simulink model "flocking_algorithm"  (R2025b)
settings: Solver=ode4  StartTime=0.0  StopTime=500  FixedStep=0.01  RelTol=1e-3
libraries: simulink_extras x9
(part 1 of 2)
settings Model: Creator=chang  LastModifiedBy=Administrator

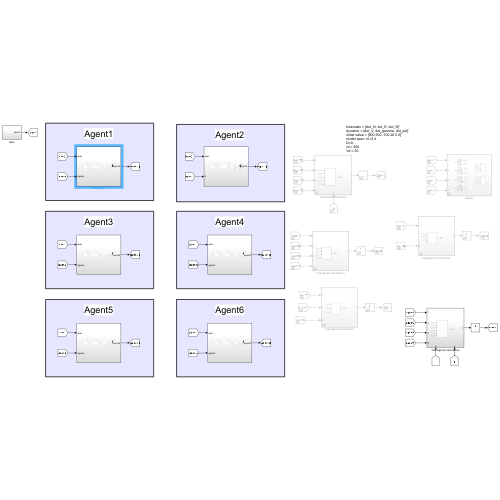
[thumbnail: Simulink's stored preview of the top-level diagram]
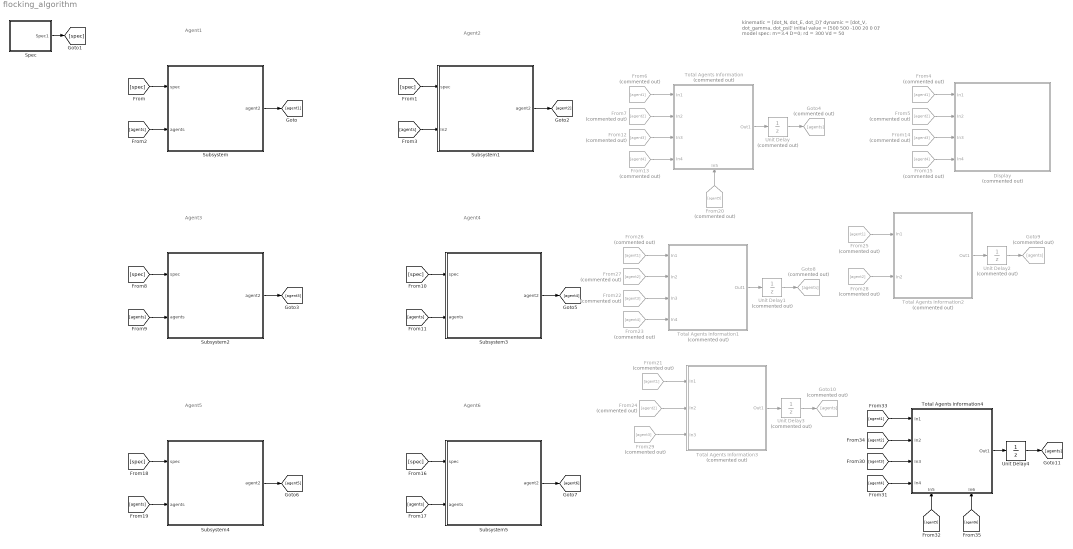
== system flocking_algorithm ==
  note: Agent1
  note: kinematic = [dot_N, dot_E, dot_D]'
      | dynamic = [dot_V, dot_gamma, dot_psi]'
      | initial value = [500 500 -100 20 0 0]'
      | model spec: m=3.4
      | D=0;
      | rd = 300
      | Vd = 50
  note: Agent2
  note: Agent3
  note: Agent4
  note: Agent5
  note: Agent6
  Display : Subsystem  Commented=on
  From{12,14,22,29} (4 alike) : From  Commented=on  GotoTag=agent3
  From13 : From  Commented=on  GotoTag=agent4
  From15 : From  Commented=on  GotoTag=agent4
  From20 : From  Commented=on  GotoTag=agent5
  From{4,6,21,25..26} (5 alike) : From  Commented=on  GotoTag=agent1
  From23 : From  Commented=on  GotoTag=agent4
  From{5,7,24,27..28} (5 alike) : From  Commented=on  GotoTag=agent2
  Goto{4,8..10} (4 alike) : Goto  Commented=on  GotoTag=agents
  Spec : Subsystem
  Subsystem : Subsystem
  Subsystem1 : Subsystem
  Subsystem2 : Subsystem
  Subsystem3 : Subsystem
  Subsystem4 : Subsystem
  Subsystem5 : Subsystem
  Total Agents Information : Subsystem  Commented=on
      settings: PortSchema="{\"entries\":[{\"content\":{\"sides\":[{\"content\":{\"connectorIds\":[\"In1\",\"In2\",\"In3\",\"In4\"]},\"type\":\"ConnectorPlacement.EquallySpacedRectSide\",\"uuid\":\"e43ed8c9-8aa1-4204-b6a6-30ae9222babf\"},{\"content\":{\"connectorIds\":[\"Out1\"],\"side\":\"RIGHT\"},\"type\":\"ConnectorPlacement.EquallySpacedRectSide\",\"uuid\":\"08aef384-d870-4c51-a80b-184b5836c24d\"},{\"content\":{\"side\":\"TOP\"},\"type\":\"ConnectorPlacement.EquallySpacedRectSide\",\"uuid\":\"5ba70bed-f88c-44da-8fba-8008d18066d7\"},{\"content\":{\"connectorIds\":[\"In5\"],\"side\":\"BOTTOM\"},\"type\":\"ConnectorPlacement.EquallySpacedRectSide\",\"uuid\":\"c2369018-f13e-4eb4-997b-0da9921f82e2\"}]},\"type\":\"ConnectorPlacement.EquallySpacedConnector\",\"uuid\":\"929a7d50-5615-46ab-b178-754a3aebd756\"}],\"packageUris\":[\"http://schema.mathworks.com/mf0/Connector/R2020b\"],\"version\":\"1.0\"}"
  Total Agents Information1 : Subsystem  Commented=on
  Total Agents Information2 : Subsystem  Commented=on
  Total Agents Information3 : Subsystem  Commented=on
  Total Agents Information4 : Subsystem
      settings: PortSchema="{\"entries\":[{\"content\":{\"sides\":[{\"content\":{\"connectorIds\":[\"In1\",\"In2\",\"In3\",\"In4\"]},\"type\":\"ConnectorPlacement.EquallySpacedRectSide\",\"uuid\":\"e43ed8c9-8aa1-4204-b6a6-30ae9222babf\"},{\"content\":{\"connectorIds\":[\"Out1\"],\"side\":\"RIGHT\"},\"type\":\"ConnectorPlacement.EquallySpacedRectSide\",\"uuid\":\"08aef384-d870-4c51-a80b-184b5836c24d\"},{\"content\":{\"side\":\"TOP\"},\"type\":\"ConnectorPlacement.EquallySpacedRectSide\",\"uuid\":\"5ba70bed-f88c-44da-8fba-8008d18066d7\"},{\"content\":{\"connectorIds\":[\"In5\",\"In6\"],\"side\":\"BOTTOM\"},\"type\":\"ConnectorPlacement.EquallySpacedRectSide\",\"uuid\":\"c2369018-f13e-4eb4-997b-0da9921f82e2\"}]},\"type\":\"ConnectorPlacement.EquallySpacedConnector\",\"uuid\":\"929a7d50-5615-46ab-b178-754a3aebd756\"}],\"packageUris\":[\"http://schema.mathworks.com/mf0/Connector/R2020b\"],\"version\":\"1.0\"}"
  Unit Delay{,1..3} (4 alike) : UnitDelay  Commented=on  SampleTime=-1  HasFrameUpgradeWarning=on
  Unit Delay4 : UnitDelay  SampleTime=-1  HasFrameUpgradeWarning=on
  wires:
  [spec] -> Subsystem/1(spec)
  [agents] -> Subsystem/2(agents)
  Subsystem1/1(agent2) -> [agent2]
  [agents] -> Subsystem1/2(In2)
  [spec] -> Subsystem1/1(spec)
  Subsystem/1(agent2) -> [agent1]
  Spec/1(Spec1) -> [spec]
  Unit Delay/1 -> Goto4/1
  From4/1 -> Display/1(In1)
  From5/1 -> Display/2(In2)
  From6/1 -> Total Agents Information/1(In1)
  From7/1 -> Total Agents Information/2(In2)
  Total Agents Information/1(Out1) -> Unit Delay/1
  [spec] -> Subsystem2/1(spec)
  [agents] -> Subsystem2/2(agents)
  Subsystem2/1(agent2) -> [agent3]
  [spec] -> Subsystem3/1(spec)
  [agents] -> Subsystem3/2(agents)
  Subsystem3/1(agent2) -> [agent4]
  From12/1 -> Total Agents Information/3(In3)
  From13/1 -> Total Agents Information/4(In4)
  From15/1 -> Display/4(In4)
  From14/1 -> Display/3(In3)
  [spec] -> Subsystem4/1(spec)
  [agents] -> Subsystem4/2(agents)
  [spec] -> Subsystem5/1(spec)
  Subsystem5/1(agent2) -> [agent6]
  [agents] -> Subsystem5/2(agents)
  Subsystem4/1(agent2) -> [agent5]
  From20/1 -> Total Agents Information/5(In5)
  Unit Delay1/1 -> Goto8/1
  From27/1 -> Total Agents Information1/2(In2)
  Total Agents Information1/1(Out1) -> Unit Delay1/1
  From26/1 -> Total Agents Information1/1(In1)
  From22/1 -> Total Agents Information1/3(In3)
  From23/1 -> Total Agents Information1/4(In4)
  From25/1 -> Total Agents Information2/1(In1)
  Unit Delay2/1 -> Goto9/1
  From28/1 -> Total Agents Information2/2(In2)
  Total Agents Information2/1(Out1) -> Unit Delay2/1
  From24/1 -> Total Agents Information3/2(In2)
  Unit Delay3/1 -> Goto10/1
  From21/1 -> Total Agents Information3/1(In1)
  Total Agents Information3/1(Out1) -> Unit Delay3/1
  From29/1 -> Total Agents Information3/3(In3)
  [agent5] -> Total Agents Information4/5(In5)
  Total Agents Information4/1(Out1) -> Unit Delay4/1
  Unit Delay4/1 -> [agents]
  [agent2] -> Total Agents Information4/2(In2)
  [agent1] -> Total Agents Information4/1(In1)
  [agent3] -> Total Agents Information4/3(In3)
  [agent4] -> Total Agents Information4/4(In4)
  [agent6] -> Total Agents Information4/6(In6)

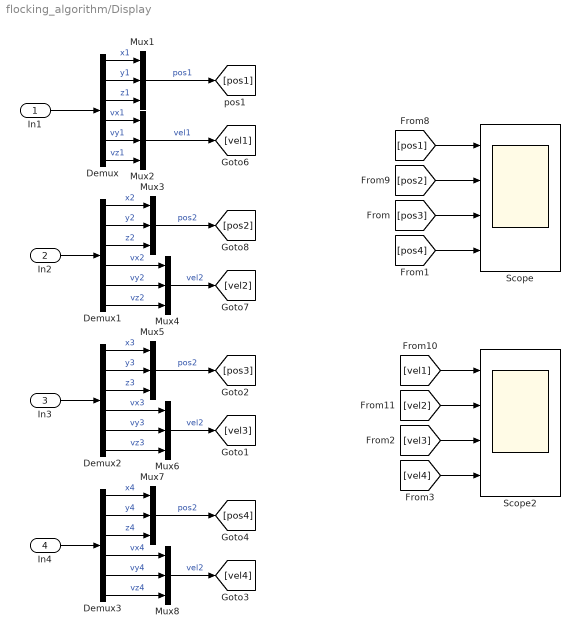
== system flocking_algorithm/Display ==
  In1 : Inport
  In2 : Inport  Port=2
  In3 : Inport  Port=3
  In4 : Inport  Port=4
  Demux{,1..3} (4 alike) : Demux  Outputs=6
  Mux{1..8} (8 alike) : Mux  Inputs=3
  Scope : Scope  NumInputPorts=4
      settings: ActiveDisplayYMinimum=-791.01816561476244  ActiveDisplayYMaximum=1093.5677488237882
  Scope2 : Scope  NumInputPorts=4
      settings: ActiveDisplayYMinimum=-365.07848233983896  ActiveDisplayYMaximum=72.840870211825987  DataLoggingVariableName=ScopeData7
  wires:
  Mux3/1 -> [pos2]  "pos2"
  Demux1/4 -> Mux4/1  "vx2"
  [pos2] -> Scope/2
  Demux/6 -> Mux2/3  "vz1"
  Demux/1 -> Mux1/1  "x1"
  Demux/4 -> Mux2/1  "vx1"
  Demux1/5 -> Mux4/2  "vy2"
  Mux2/1 -> [vel1]  "vel1"
  [vel1] -> Scope2/1
  Demux1/2 -> Mux3/2  "y2"
  Demux/3 -> Mux1/3  "z1"
  Demux/2 -> Mux1/2  "y1"
  Demux1/1 -> Mux3/1  "x2"
  Demux1/3 -> Mux3/3  "z2"
  [pos1] -> Scope/1
  Mux4/1 -> [vel2]  "vel2"
  Demux1/6 -> Mux4/3  "vz2"
  Mux1/1 -> [pos1]  "pos1"
  Demux/5 -> Mux2/2  "vy1"
  [vel2] -> Scope2/2
  In2/1 -> Demux1/1
  In1/1 -> Demux/1
  Demux2/5 -> Mux6/2  "vy3"
  Demux2/6 -> Mux6/3  "vz3"
  Demux2/4 -> Mux6/1  "vx3"
  Mux5/1 -> [pos3]  "pos2"
  In3/1 -> Demux2/1
  Demux2/3 -> Mux5/3  "z3"
  Mux6/1 -> [vel3]  "vel2"
  Demux2/1 -> Mux5/1  "x3"
  Demux2/2 -> Mux5/2  "y3"
  Demux3/5 -> Mux8/2  "vy4"
  Demux3/6 -> Mux8/3  "vz4"
  Demux3/4 -> Mux8/1  "vx4"
  Mux7/1 -> [pos4]  "pos2"
  In4/1 -> Demux3/1
  Demux3/3 -> Mux7/3  "z4"
  Mux8/1 -> [vel4]  "vel2"
  Demux3/1 -> Mux7/1  "x4"
  Demux3/2 -> Mux7/2  "y4"
  [pos3] -> Scope/3
  [pos4] -> Scope/4
  [vel3] -> Scope2/3
  [vel4] -> Scope2/4

== system flocking_algorithm/Spec ==
  Spec : Subsystem
  Spec1 : Outport
  wires:
  Spec/1(Spec) -> Spec1/1

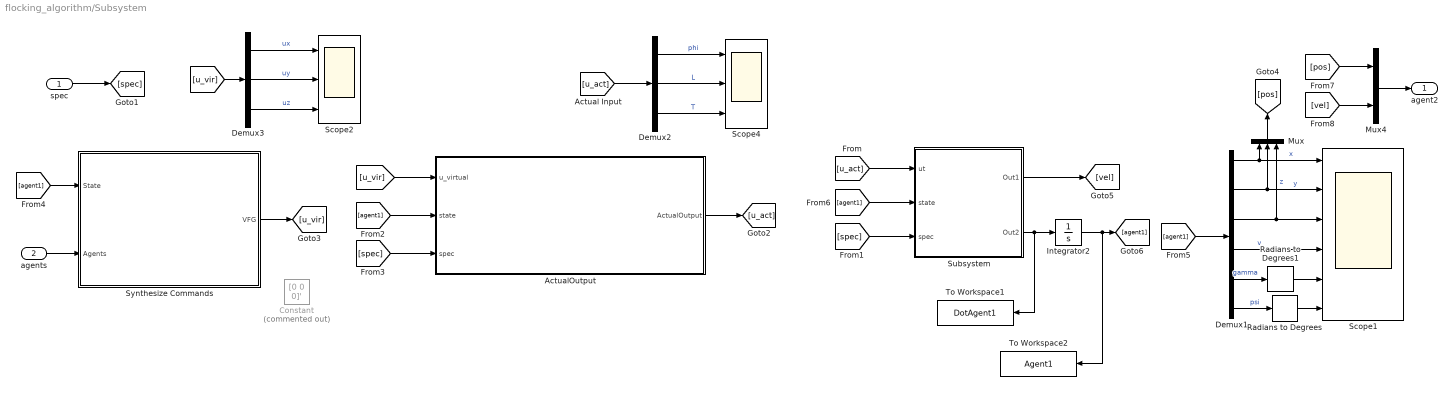
== system flocking_algorithm/Subsystem ==
  spec : Inport
  agents : Inport  Port=2
  ActualOutput : Subsystem
  Constant : Constant  Commented=on  Value=[0 0 0]'
  Demux1 : Demux  Outputs=6
  Demux2 : Demux  Outputs=3
  Demux3 : Demux  Outputs=3
  Integrator2 : Integrator  InitialCondition=[-1800 2000 -100 20 0 0]'  UpperSaturationLimit=[10^6 ;10^6 ;10^6 ;30 ;15 ;10^6]  LowerSaturationLimit=[-10^6; -10^6 ;-10^6; 0; -15 ;-10^6]'
  Mux : Mux  Inputs=3
  Mux4 : Mux  Inputs=2
  Radians to Degrees : simulink_extras/Transformations/Radians to Degrees
  Radians to Degrees1 : simulink_extras/Transformations/Radians to Degrees
  Scope1 : Scope  NumInputPorts=6
      settings: ActiveDisplayYMinimum=-1.7966158577892821E+72  ActiveDisplayYMaximum=1.5570735154634757E+73  DataLoggingVariableName=ScopeData3
  Scope2 : Scope  NumInputPorts=3
      settings: ActiveDisplayYMinimum=-5.0247050713987121E+98  ActiveDisplayYMaximum=6.7419493762501636E+97
  Scope4 : Scope  NumInputPorts=3
      settings: ActiveDisplayYMinimum=-3.9266304802667316  ActiveDisplayYMaximum=3.9246740137432026  DataLoggingVariableName=ScopeData5
  Subsystem : Subsystem
  Synthesize Commands : Subsystem
  To Workspace1 : ToWorkspace  VariableName=DotAgent1  SaveFormat=Timeseries  SampleTime=-1
  To Workspace2 : ToWorkspace  VariableName=Agent1  SaveFormat=Timeseries  SampleTime=-1
  agent2 : Outport
  wires:
  [agent1] -> ActualOutput/2(state)
  Demux1/3 -> Mux/3, Scope1/3  "z"
  Demux1/4 -> Scope1/4  "v"
  Demux1/1 -> Mux/1, Scope1/1  "x"
  [spec] -> ActualOutput/3(spec)
  Demux2/1 -> Scope4/1  "phi"
  Demux2/3 -> Scope4/3  "T"
  Demux1/2 -> Mux/2, Scope1/2  "y"
  Demux2/2 -> Scope4/2  "L"
  [u_vir] -> Demux3/1
  [agent1] -> Demux1/1
  Demux1/5 -> Radians to Degrees1/1  "gamma"
  Demux1/6 -> Radians to Degrees/1  "psi"
  [u_act] -> Demux2/1
  Demux3/2 -> Scope2/2  "uy"
  Demux3/1 -> Scope2/1  "ux"
  Demux3/3 -> Scope2/3  "uz"
  [u_vir] -> ActualOutput/1(u_virtual)
  spec/1 -> [spec]
  Mux/1 -> [pos]
  Integrator2/1 -> [agent1], To Workspace2/1
  Mux4/1 -> agent2/1
  [vel] -> Mux4/2
  [pos] -> Mux4/1
  [agent1] -> Synthesize Commands/1(State)
  agents/1 -> Synthesize Commands/2(Agents)
  [u_act] -> Subsystem/1(ut)
  [agent1] -> Subsystem/2(state)
  [spec] -> Subsystem/3(spec)
  Subsystem/1(Out1) -> [vel]
  Subsystem/2(Out2) -> To Workspace1/1, Integrator2/1
  Synthesize Commands/1(VFG) -> [u_vir]
  ActualOutput/1(ActualOutput) -> [u_act]
  Radians to Degrees/1 -> Scope1/6
  Radians to Degrees1/1 -> Scope1/5

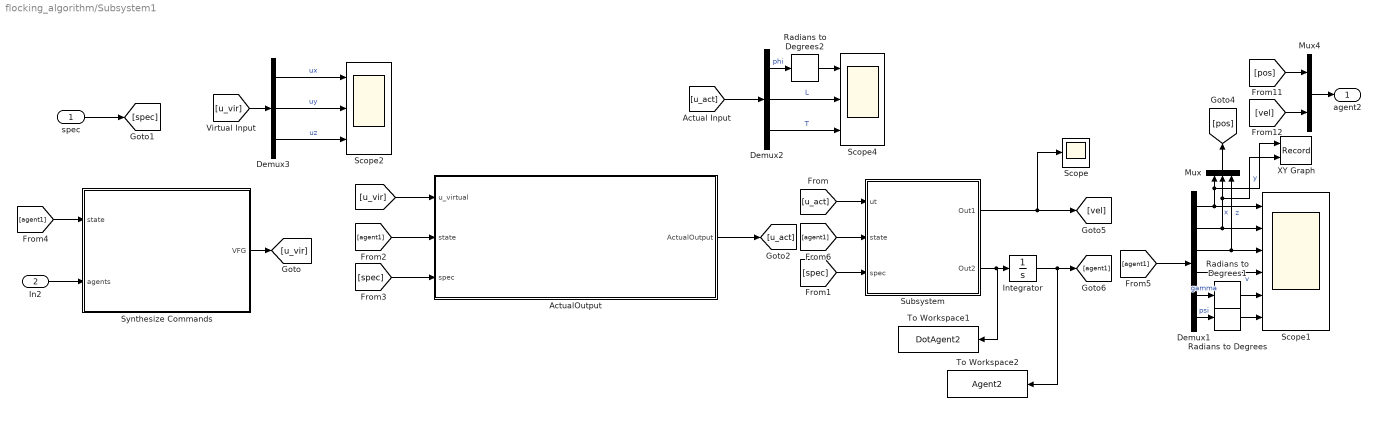
== system flocking_algorithm/Subsystem1 ==
  spec : Inport
  In2 : Inport  Port=2
  ActualOutput : Subsystem
  Demux1 : Demux  Outputs=6
  Demux2 : Demux  Outputs=3
  Demux3 : Demux  Outputs=3
  Integrator : Integrator  InitialCondition=[2000 1800 -100 20 0 0]'
  Mux : Mux  Inputs=3
  Mux4 : Mux  Inputs=2
  Radians to Degrees : simulink_extras/Transformations/Radians to Degrees
  Radians to Degrees1 : simulink_extras/Transformations/Radians to Degrees
  Radians to Degrees2 : simulink_extras/Transformations/Radians to Degrees
  Scope : Scope
      settings: ActiveDisplayYMinimum=-24.999999982546566  ActiveDisplayYMaximum=24.99999999806073  DataLoggingVariableName=ScopeData9
  Scope1 : Scope  NumInputPorts=6
      settings: ActiveDisplayYMinimum=-752.136140008936  ActiveDisplayYMaximum=1201.12192036178  DataLoggingVariableName=ScopeData3
  Scope2 : Scope  NumInputPorts=3
      settings: ActiveDisplayYMinimum=-50.131614103473233  ActiveDisplayYMaximum=7.8433072052775152
  Scope4 : Scope  NumInputPorts=3
      settings: ActiveDisplayYMinimum=-114.79277060053131  ActiveDisplayYMaximum=208.28266105424055  DataLoggingVariableName=ScopeData5
  Subsystem : Subsystem
  Synthesize Commands : Subsystem
  To Workspace1 : ToWorkspace  VariableName=DotAgent2  SaveFormat=Timeseries  SampleTime=-1
  To Workspace2 : ToWorkspace  VariableName=Agent2  SaveFormat=Timeseries  SampleTime=-1
  XY Graph : Record  NumPorts=2.0  FileSettingsInternal="{\"entries\":[{\"content\":{\"excelSettings\":{\"content\":{},\"type\":\"Streamout.ExcelSettings\"},\"parquetSettings\":{\"content\":{},\"type\":\"Streamout.ParquetSettings\"}},\"type\":\"Streamout.FileSettingStorage\",\"uuid\":\"\"}],\"packageUris\":[\"http:\\/\\/schema.mathworks.com\\/mf0\\/streamout_blocks\\/R2020a\"],\"version\":\"1.0\"}"  FrameSettings=[0, 0]  Layout=[1 1]  SignalsInternal="{\"entries\":[{\"content\":{\"signals\":[{\"content\":{\"blockPath\":[],\"dimensions\":[1],\"domain\":\"\",\"lineColor\":\"#a2142f\",\"plots\":[ 1 ],\"port\":1,\"signalID\":1,\"signalName\":\"x\"},\"type\":\"RecordBlkView.Signal\",\"uuid\":\"\"},{\"content\":{\"blockPath\":[],\"dimensions\":[1],\"domain\":\"\",\"lineColor\":\"#139fff\",\"plots\":[ 1 ],\"port\":2,\"signalID\":2,\"signalName\":\"y\"},\"type\":\"RecordBlkView.Signal\",\"uuid\":\"\"}]},\"type\":\"RecordBlkView.InputSignals\",\"uuid\":\"\"}],\"packageUris\":[\"http:\\/\\/schema.mathworks.com\\/mf0\\/streamout_blocks\\/R2020a\"],\"version\":\"1.0\"}"  VisualizationBindings="{\"xyplotplugin\":{\"info\":[{\"series\":[{\"bindingParametersList\":[{\"parameter\":\"X-Axis\",\"signalID\":1,\"signalName\":\"x\"},{\"parameter\":\"Y-Axis\",\"signalID\":2,\"signalName\":\"y\"}],\"seriesID\":0}],\"subplotID\":1}]}}"  CompatibilityTag=XY
  agent2 : Outport
  wires:
  [agent1] -> ActualOutput/2(state)
  Demux1/3 -> Scope1/3, Mux/3  "z"
  Demux1/4 -> Scope1/4  "v"
  Demux1/1 -> Scope1/1, XY Graph/1, Mux/1  "x"
  [spec] -> ActualOutput/3(spec)
  ActualOutput/1(ActualOutput) -> [u_act]
  Demux2/1 -> Radians to Degrees2/1  "phi"
  Demux2/3 -> Scope4/3  "T"
  Demux1/2 -> Scope1/2, XY Graph/2, Mux/2  "y"
  Demux2/2 -> Scope4/2  "L"
  [u_vir] -> Demux3/1
  [agent1] -> Demux1/1
  Demux1/5 -> Radians to Degrees1/1  "gamma"
  Demux1/6 -> Radians to Degrees/1  "psi"
  [u_act] -> Demux2/1
  Demux3/2 -> Scope2/2  "uy"
  Demux3/1 -> Scope2/1  "ux"
  Demux3/3 -> Scope2/3  "uz"
  [u_vir] -> ActualOutput/1(u_virtual)
  spec/1 -> [spec]
  Mux/1 -> [pos]
  [pos] -> Mux4/1
  [vel] -> Mux4/2
  Mux4/1 -> agent2/1
  Subsystem/2(Out2) -> To Workspace1/1, Integrator/1
  [agent1] -> Synthesize Commands/1(state)
  Synthesize Commands/1(VFG) -> [u_vir]
  [u_act] -> Subsystem/1(ut)
  [agent1] -> Subsystem/2(state)
  [spec] -> Subsystem/3(spec)
  Subsystem/1(Out1) -> Scope/1, [vel]
  Radians to Degrees/1 -> Scope1/6
  Radians to Degrees1/1 -> Scope1/5
  Radians to Degrees2/1 -> Scope4/1
  In2/1 -> Synthesize Commands/2(agents)
  Integrator/1 -> [agent1], To Workspace2/1

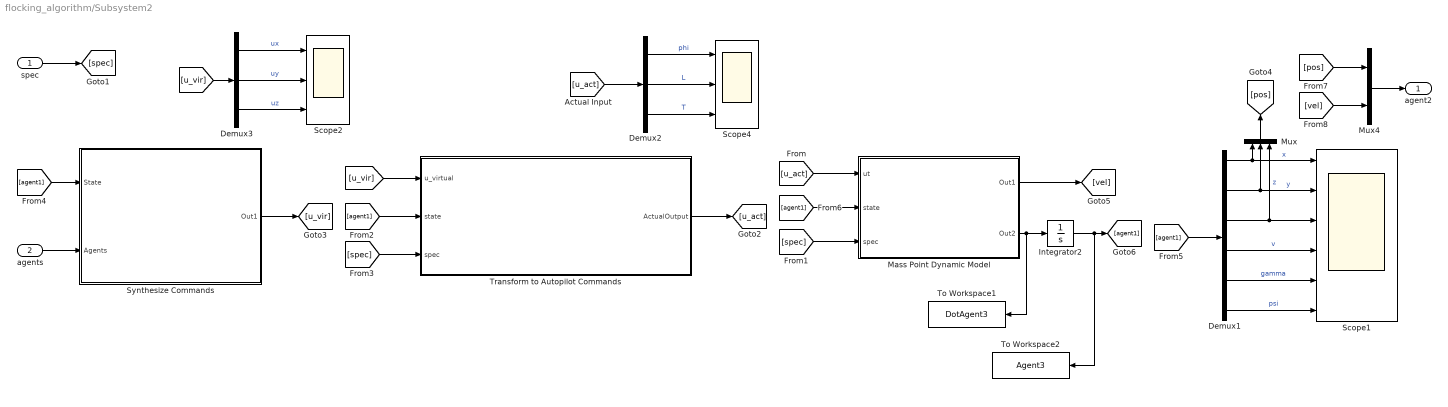
== system flocking_algorithm/Subsystem2 ==
  spec : Inport
  agents : Inport  Port=2
  Demux1 : Demux  Outputs=6
  Demux2 : Demux  Outputs=3
  Demux3 : Demux  Outputs=3
  Integrator2 : Integrator  InitialCondition=[800 -900 -100 20 0 0]'  UpperSaturationLimit=[10^6; 10^6 ;10^6; 30; 15 ;10^6]'  LowerSaturationLimit=[-10^6; -10^6 ;-10^6; 0; -15 ;-10^6]'
  Mass Point Dynamic Model : Subsystem
  Mux : Mux  Inputs=3
  Mux4 : Mux  Inputs=2
  Scope1 : Scope  NumInputPorts=6
      settings: ActiveDisplayYMinimum=-754.5317420687536  ActiveDisplayYMaximum=1100.6939107466712  DataLoggingVariableName=ScopeData3
  Scope2 : Scope  NumInputPorts=3
      settings: ActiveDisplayYMinimum=-43.390695181246379  ActiveDisplayYMaximum=10.376743909027375
  Scope4 : Scope  NumInputPorts=3
      settings: ActiveDisplayYMinimum=-0.43593009457122217  ActiveDisplayYMaximum=1.7820174500860297  DataLoggingVariableName=ScopeData5
  Synthesize Commands : Subsystem
  To Workspace1 : ToWorkspace  VariableName=DotAgent3  SaveFormat=Timeseries  SampleTime=-1
  To Workspace2 : ToWorkspace  VariableName=Agent3  SaveFormat=Timeseries  SampleTime=-1
  Transform to Autopilot Commands : Subsystem
  agent2 : Outport
  wires:
  [agent1] -> Transform to Autopilot Commands/2(state)
  Demux1/3 -> Mux/3, Scope1/3  "z"
  Demux1/4 -> Scope1/4  "v"
  Demux1/1 -> Mux/1, Scope1/1  "x"
  [spec] -> Transform to Autopilot Commands/3(spec)
  Transform to Autopilot Commands/1(ActualOutput) -> [u_act]
  Demux2/1 -> Scope4/1  "phi"
  Demux2/3 -> Scope4/3  "T"
  Demux1/2 -> Mux/2, Scope1/2  "y"
  Demux2/2 -> Scope4/2  "L"
  [u_vir] -> Demux3/1
  [agent1] -> Demux1/1
  Demux1/5 -> Scope1/5  "gamma"
  Demux1/6 -> Scope1/6  "psi"
  [u_act] -> Demux2/1
  Demux3/2 -> Scope2/2  "uy"
  Demux3/1 -> Scope2/1  "ux"
  Demux3/3 -> Scope2/3  "uz"
  [u_vir] -> Transform to Autopilot Commands/1(u_virtual)
  spec/1 -> [spec]
  Mux/1 -> [pos]
  Integrator2/1 -> [agent1], To Workspace2/1
  Mux4/1 -> agent2/1
  [vel] -> Mux4/2
  [pos] -> Mux4/1
  [agent1] -> Synthesize Commands/1(State)
  agents/1 -> Synthesize Commands/2(Agents)
  Synthesize Commands/1(Out1) -> [u_vir]
  [u_act] -> Mass Point Dynamic Model/1(ut)
  [agent1] -> Mass Point Dynamic Model/2(state)
  [spec] -> Mass Point Dynamic Model/3(spec)
  Mass Point Dynamic Model/1(Out1) -> [vel]
  Mass Point Dynamic Model/2(Out2) -> To Workspace1/1, Integrator2/1

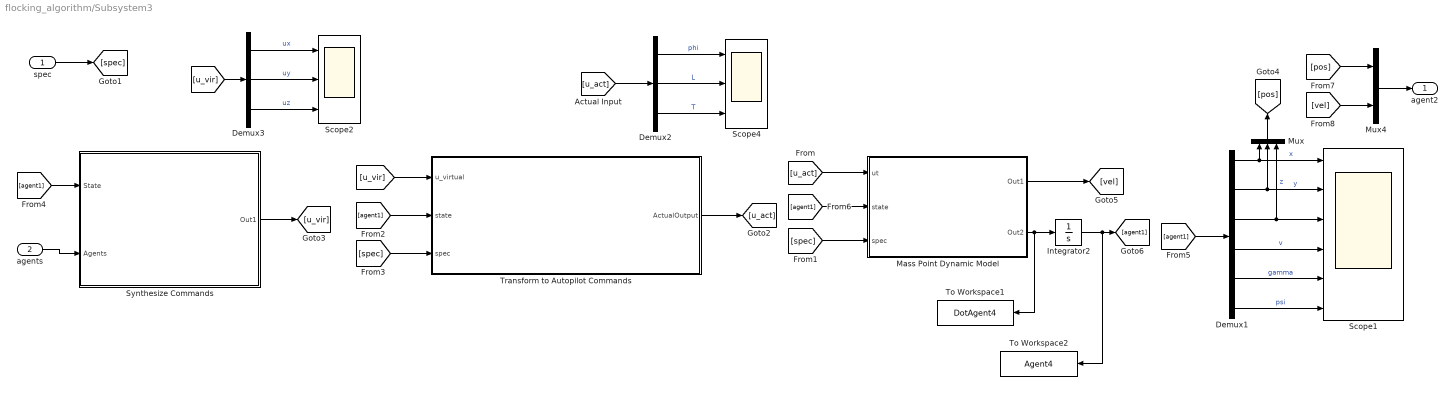
== system flocking_algorithm/Subsystem3 ==
  spec : Inport
  agents : Inport  Port=2
  Demux1 : Demux  Outputs=6
  Demux2 : Demux  Outputs=3
  Demux3 : Demux  Outputs=3
  Integrator2 : Integrator  InitialCondition=[900 -1000 -100 20 0 0]'  UpperSaturationLimit=[10^6;10^6 ;10^6; 30; 15 ;10^6]'  LowerSaturationLimit=[-10^6; -10^6 ;-10^6; 0; -15 ;-10^6]'
  Mass Point Dynamic Model : Subsystem
  Mux : Mux  Inputs=3
  Mux4 : Mux  Inputs=2
  Scope1 : Scope  NumInputPorts=6
      settings: ActiveDisplayYMinimum=-775.24470531151951  ActiveDisplayYMaximum=1094.5034869964145  DataLoggingVariableName=ScopeData3
  Scope2 : Scope  NumInputPorts=3
      settings: ActiveDisplayYMinimum=-50.976263436423132  ActiveDisplayYMaximum=27.271065899369784
  Scope4 : Scope  NumInputPorts=3
      settings: ActiveDisplayYMinimum=-1.6818846962105793  ActiveDisplayYMaximum=0.93255510942344089  DataLoggingVariableName=ScopeData5
  Synthesize Commands : Subsystem
  To Workspace1 : ToWorkspace  VariableName=DotAgent4  SaveFormat=Timeseries  SampleTime=-1
  To Workspace2 : ToWorkspace  VariableName=Agent4  SaveFormat=Timeseries  SampleTime=-1
  Transform to Autopilot Commands : Subsystem
  agent2 : Outport
  wires:
  [agent1] -> Transform to Autopilot Commands/2(state)
  Demux1/3 -> Mux/3, Scope1/3  "z"
  Demux1/4 -> Scope1/4  "v"
  Demux1/1 -> Mux/1, Scope1/1  "x"
  [spec] -> Transform to Autopilot Commands/3(spec)
  Transform to Autopilot Commands/1(ActualOutput) -> [u_act]
  Demux2/1 -> Scope4/1  "phi"
  Demux2/3 -> Scope4/3  "T"
  Demux1/2 -> Mux/2, Scope1/2  "y"
  Demux2/2 -> Scope4/2  "L"
  [u_vir] -> Demux3/1
  [agent1] -> Demux1/1
  Demux1/5 -> Scope1/5  "gamma"
  Demux1/6 -> Scope1/6  "psi"
  [u_act] -> Demux2/1
  Demux3/2 -> Scope2/2  "uy"
  Demux3/1 -> Scope2/1  "ux"
  Demux3/3 -> Scope2/3  "uz"
  [u_vir] -> Transform to Autopilot Commands/1(u_virtual)
  spec/1 -> [spec]
  Mux/1 -> [pos]
  Integrator2/1 -> [agent1], To Workspace2/1
  Mux4/1 -> agent2/1
  [vel] -> Mux4/2
  [pos] -> Mux4/1
  [agent1] -> Synthesize Commands/1(State)
  agents/1 -> Synthesize Commands/2(Agents)
  Synthesize Commands/1(Out1) -> [u_vir]
  [u_act] -> Mass Point Dynamic Model/1(ut)
  [agent1] -> Mass Point Dynamic Model/2(state)
  [spec] -> Mass Point Dynamic Model/3(spec)
  Mass Point Dynamic Model/1(Out1) -> [vel]
  Mass Point Dynamic Model/2(Out2) -> To Workspace1/1, Integrator2/1

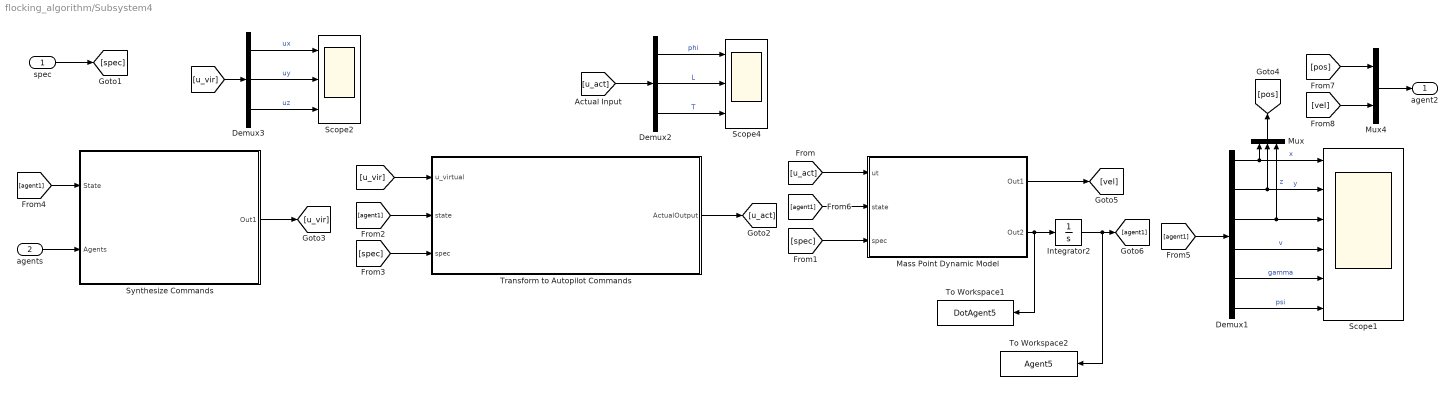
== system flocking_algorithm/Subsystem4 ==
  spec : Inport
  agents : Inport  Port=2
  Demux1 : Demux  Outputs=6
  Demux2 : Demux  Outputs=3
  Demux3 : Demux  Outputs=3
  Integrator2 : Integrator  InitialCondition=[-800 -800 -100 20 0 0]'
  Mass Point Dynamic Model : Subsystem
  Mux : Mux  Inputs=3
  Mux4 : Mux  Inputs=2
  Scope1 : Scope  NumInputPorts=6
      settings: ActiveDisplayYMinimum=-754.5317420687536  ActiveDisplayYMaximum=1100.6939107466712  DataLoggingVariableName=ScopeData3
  Scope2 : Scope  NumInputPorts=3
      settings: ActiveDisplayYMinimum=-43.390695181246379  ActiveDisplayYMaximum=10.376743909027375
  Scope4 : Scope  NumInputPorts=3
      settings: ActiveDisplayYMinimum=-0.43593009457122217  ActiveDisplayYMaximum=1.7820174500860297  DataLoggingVariableName=ScopeData5
  Synthesize Commands : Subsystem
  To Workspace1 : ToWorkspace  VariableName=DotAgent5  SaveFormat=Timeseries  SampleTime=-1
  To Workspace2 : ToWorkspace  VariableName=Agent5  SaveFormat=Timeseries  SampleTime=-1
  Transform to Autopilot Commands : Subsystem
  agent2 : Outport
  wires:
  [agent1] -> Transform to Autopilot Commands/2(state)
  Demux1/3 -> Mux/3, Scope1/3  "z"
  Demux1/4 -> Scope1/4  "v"
  Demux1/1 -> Mux/1, Scope1/1  "x"
  [spec] -> Transform to Autopilot Commands/3(spec)
  Transform to Autopilot Commands/1(ActualOutput) -> [u_act]
  Demux2/1 -> Scope4/1  "phi"
  Demux2/3 -> Scope4/3  "T"
  Demux1/2 -> Mux/2, Scope1/2  "y"
  Demux2/2 -> Scope4/2  "L"
  [u_vir] -> Demux3/1
  [agent1] -> Demux1/1
  Demux1/5 -> Scope1/5  "gamma"
  Demux1/6 -> Scope1/6  "psi"
  [u_act] -> Demux2/1
  Demux3/2 -> Scope2/2  "uy"
  Demux3/1 -> Scope2/1  "ux"
  Demux3/3 -> Scope2/3  "uz"
  [u_vir] -> Transform to Autopilot Commands/1(u_virtual)
  spec/1 -> [spec]
  Mux/1 -> [pos]
  Integrator2/1 -> [agent1], To Workspace2/1
  Mux4/1 -> agent2/1
  [vel] -> Mux4/2
  [pos] -> Mux4/1
  [agent1] -> Synthesize Commands/1(State)
  agents/1 -> Synthesize Commands/2(Agents)
  Synthesize Commands/1(Out1) -> [u_vir]
  [u_act] -> Mass Point Dynamic Model/1(ut)
  [agent1] -> Mass Point Dynamic Model/2(state)
  [spec] -> Mass Point Dynamic Model/3(spec)
  Mass Point Dynamic Model/1(Out1) -> [vel]
  Mass Point Dynamic Model/2(Out2) -> To Workspace1/1, Integrator2/1

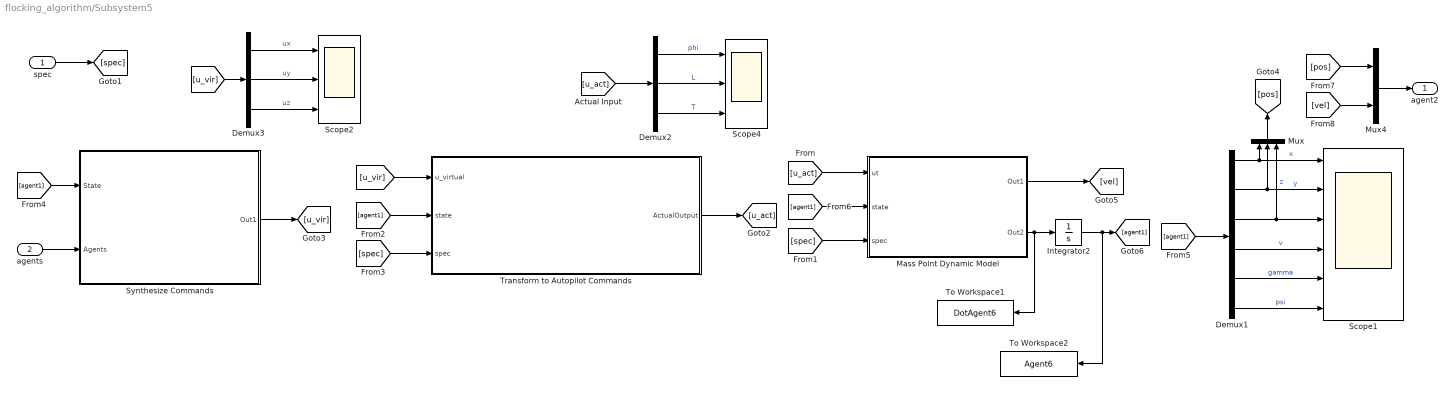
== system flocking_algorithm/Subsystem5 ==
  spec : Inport
  agents : Inport  Port=2
  Demux1 : Demux  Outputs=6
  Demux2 : Demux  Outputs=3
  Demux3 : Demux  Outputs=3
  Integrator2 : Integrator  InitialCondition=[800 -900 -100 20 0 0]'
  Mass Point Dynamic Model : Subsystem
  Mux : Mux  Inputs=3
  Mux4 : Mux  Inputs=2
  Scope1 : Scope  NumInputPorts=6
      settings: ActiveDisplayYMinimum=-694.81081921046984  ActiveDisplayYMaximum=1103.0528933392313  DataLoggingVariableName=ScopeData3
  Scope2 : Scope  NumInputPorts=3
      settings: ActiveDisplayYMinimum=-43.390695181246379  ActiveDisplayYMaximum=10.376743909027375
  Scope4 : Scope  NumInputPorts=3
      settings: ActiveDisplayYMinimum=-1.6818846962105793  ActiveDisplayYMaximum=0.93255510942344089  DataLoggingVariableName=ScopeData5
  Synthesize Commands : Subsystem
  To Workspace1 : ToWorkspace  VariableName=DotAgent6  SaveFormat=Timeseries  SampleTime=-1
  To Workspace2 : ToWorkspace  VariableName=Agent6  SaveFormat=Timeseries  SampleTime=-1
  Transform to Autopilot Commands : Subsystem
  agent2 : Outport
  wires:
  [agent1] -> Transform to Autopilot Commands/2(state)
  Demux1/3 -> Mux/3, Scope1/3  "z"
  Demux1/4 -> Scope1/4  "v"
  Demux1/1 -> Mux/1, Scope1/1  "x"
  [spec] -> Transform to Autopilot Commands/3(spec)
  Transform to Autopilot Commands/1(ActualOutput) -> [u_act]
  Demux2/1 -> Scope4/1  "phi"
  Demux2/3 -> Scope4/3  "T"
  Demux1/2 -> Mux/2, Scope1/2  "y"
  Demux2/2 -> Scope4/2  "L"
  [u_vir] -> Demux3/1
  [agent1] -> Demux1/1
  Demux1/5 -> Scope1/5  "gamma"
  Demux1/6 -> Scope1/6  "psi"
  [u_act] -> Demux2/1
  Demux3/2 -> Scope2/2  "uy"
  Demux3/1 -> Scope2/1  "ux"
  Demux3/3 -> Scope2/3  "uz"
  [u_vir] -> Transform to Autopilot Commands/1(u_virtual)
  spec/1 -> [spec]
  Mux/1 -> [pos]
  Integrator2/1 -> [agent1], To Workspace2/1
  Mux4/1 -> agent2/1
  [vel] -> Mux4/2
  [pos] -> Mux4/1
  [agent1] -> Synthesize Commands/1(State)
  agents/1 -> Synthesize Commands/2(Agents)
  Synthesize Commands/1(Out1) -> [u_vir]
  [u_act] -> Mass Point Dynamic Model/1(ut)
  [agent1] -> Mass Point Dynamic Model/2(state)
  [spec] -> Mass Point Dynamic Model/3(spec)
  Mass Point Dynamic Model/1(Out1) -> [vel]
  Mass Point Dynamic Model/2(Out2) -> To Workspace1/1, Integrator2/1

== system flocking_algorithm/Total Agents Information ==
  note: agents = [pos, vel ; pos, vel] = R^6X2
  In1 : Inport
  In2 : Inport  Port=2
  In3 : Inport  Port=3
  In4 : Inport  Port=4
  In5 : Inport  Port=5
  Matrix Concatenate : Concatenate  NumInputs=5  Mode=Multidimensional array  ConcatenateDimension=2
  Out1 : Outport
  wires:
  In2/1 -> Matrix Concatenate/2
  In1/1 -> Matrix Concatenate/1
  Matrix Concatenate/1 -> Out1/1
  In3/1 -> Matrix Concatenate/3
  In4/1 -> Matrix Concatenate/4
  In5/1 -> Matrix Concatenate/5

== system flocking_algorithm/Total Agents Information1 ==
  note: agents = [pos, vel ; pos, vel] = R^6X2
  In1 : Inport
  In2 : Inport  Port=2
  In3 : Inport  Port=3
  In4 : Inport  Port=4
  Matrix Concatenate : Concatenate  NumInputs=4  Mode=Multidimensional array  ConcatenateDimension=2
  Out1 : Outport
  wires:
  In2/1 -> Matrix Concatenate/2
  In1/1 -> Matrix Concatenate/1
  Matrix Concatenate/1 -> Out1/1
  In3/1 -> Matrix Concatenate/3
  In4/1 -> Matrix Concatenate/4

== system flocking_algorithm/Total Agents Information2 ==
  note: agents = [pos, vel ; pos, vel] = R^6X2
  In1 : Inport
  In2 : Inport  Port=2
  Matrix Concatenate : Concatenate  Mode=Multidimensional array  ConcatenateDimension=2
  Out1 : Outport
  wires:
  In2/1 -> Matrix Concatenate/2
  In1/1 -> Matrix Concatenate/1
  Matrix Concatenate/1 -> Out1/1

== system flocking_algorithm/Total Agents Information3 ==
  note: agents = [pos, vel ; pos, vel] = R^6X2
  In1 : Inport
  In2 : Inport  Port=2
  In3 : Inport  Port=3
  Matrix Concatenate : Concatenate  NumInputs=3  Mode=Multidimensional array  ConcatenateDimension=2
  Out1 : Outport
  wires:
  In2/1 -> Matrix Concatenate/2
  In1/1 -> Matrix Concatenate/1
  Matrix Concatenate/1 -> Out1/1
  In3/1 -> Matrix Concatenate/3

== system flocking_algorithm/Total Agents Information4 ==
  note: agents = [pos, vel ; pos, vel] = R^6X2
  In1 : Inport
  In2 : Inport  Port=2
  In3 : Inport  Port=3
  In4 : Inport  Port=4
  In5 : Inport  Port=5
  In6 : Inport  Port=6
  Matrix Concatenate : Concatenate  NumInputs=6  Mode=Multidimensional array  ConcatenateDimension=2
  Out1 : Outport
  wires:
  In2/1 -> Matrix Concatenate/2
  In1/1 -> Matrix Concatenate/1
  Matrix Concatenate/1 -> Out1/1
  In3/1 -> Matrix Concatenate/3
  In4/1 -> Matrix Concatenate/4
  In5/1 -> Matrix Concatenate/5
  In6/1 -> Matrix Concatenate/6

== system flocking_algorithm/Spec/Spec ==
  Constant3 : Constant  Value=[15 9.0806]'
  Spec : Outport
  wires:
  Constant3/1 -> Spec/1

== system flocking_algorithm/Subsystem/ActualOutput ==
  u_virtual : Inport
  state : Inport  Port=2
  spec : Inport  Port=3
  MATLAB Function : MATLAB Function  TreatAsAtomicUnit=on
  ActualOutput : Outport
  wires:
  u_virtual/1 -> MATLAB Function/1(u_virtual)
  state/1 -> MATLAB Function/2(state)
  spec/1 -> MATLAB Function/3(spec)
  MATLAB Function/1(act_out) -> ActualOutput/1

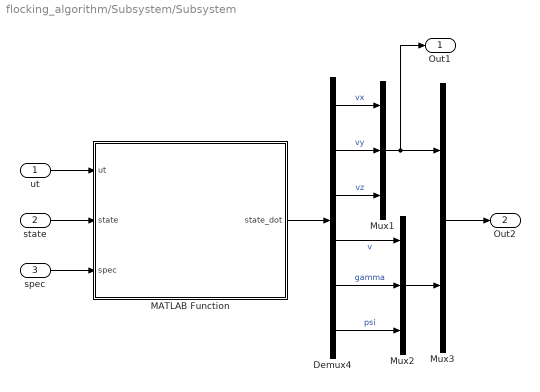
== system flocking_algorithm/Subsystem/Subsystem ==
  ut : Inport
  state : Inport  Port=2
  spec : Inport  Port=3
  Demux4 : Demux  Outputs=6
  MATLAB Function : MATLAB Function  TreatAsAtomicUnit=on
  Mux1 : Mux  Inputs=3
  Mux2 : Mux  Inputs=3
  Mux3 : Mux  Inputs=2
  Out1 : Outport
  Out2 : Outport  Port=2
  wires:
  Demux4/4 -> Mux2/1  "v"
  Demux4/2 -> Mux1/2  "vy"
  Mux1/1 -> Out1/1, Mux3/1
  Demux4/5 -> Mux2/2  "gamma"
  Demux4/3 -> Mux1/3  "vz"
  ut/1 -> MATLAB Function/1(ut)
  Mux2/1 -> Mux3/2
  Demux4/1 -> Mux1/1  "vx"
  Mux3/1 -> Out2/1
  Demux4/6 -> Mux2/3  "psi"
  MATLAB Function/1(state_dot) -> Demux4/1
  spec/1 -> MATLAB Function/3(spec)
  state/1 -> MATLAB Function/2(state)

== system flocking_algorithm/Subsystem/Synthesize Commands ==
  State : Inport
  Agents : Inport  Port=2
  Add : Sum  Inputs=+++
  Augemented Cucker Smale Model : Subsystem
  Potential Field : Subsystem
  To Workspace : ToWorkspace  VariableName=u_acs  SaveFormat=Timeseries  SampleTime=-1
  To Workspace1 : ToWorkspace  VariableName=u_pf  SaveFormat=Timeseries  SampleTime=-1
  Vector Field Guidance2 : Subsystem
  VFG : Outport
  wires:
  Augemented Cucker Smale Model/1(ACS) -> To Workspace/1, Add/2
  State/1 -> Vector Field Guidance2/1(state)
  Potential Field/1(PF) -> Add/3, To Workspace1/1
  Agents/1 -> Potential Field/1(agent), Augemented Cucker Smale Model/1(agent)
  Vector Field Guidance2/1(VFG) -> Add/1
  Add/1 -> VFG/1

== system flocking_algorithm/Subsystem1/ActualOutput ==
  u_virtual : Inport
  state : Inport  Port=2
  spec : Inport  Port=3
  MATLAB Function : MATLAB Function  TreatAsAtomicUnit=on
  ActualOutput : Outport
  wires:
  u_virtual/1 -> MATLAB Function/1(u_virtual)
  state/1 -> MATLAB Function/2(state)
  spec/1 -> MATLAB Function/3(spec)
  MATLAB Function/1(act_out) -> ActualOutput/1

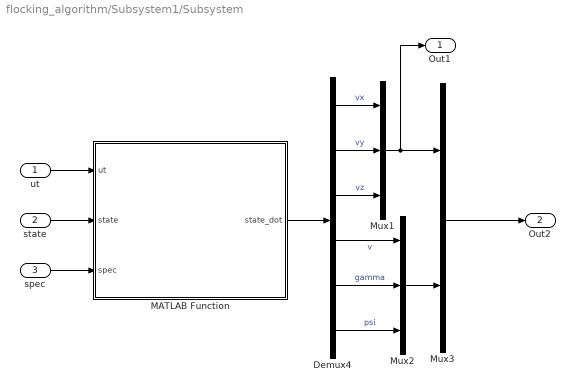
== system flocking_algorithm/Subsystem1/Subsystem ==
  ut : Inport
  state : Inport  Port=2
  spec : Inport  Port=3
  Demux4 : Demux  Outputs=6
  MATLAB Function : MATLAB Function  TreatAsAtomicUnit=on
  Mux1 : Mux  Inputs=3
  Mux2 : Mux  Inputs=3
  Mux3 : Mux  Inputs=2
  Out1 : Outport
  Out2 : Outport  Port=2
  wires:
  Demux4/4 -> Mux2/1  "v"
  Demux4/2 -> Mux1/2  "vy"
  Mux1/1 -> Out1/1, Mux3/1
  Demux4/5 -> Mux2/2  "gamma"
  Demux4/3 -> Mux1/3  "vz"
  ut/1 -> MATLAB Function/1(ut)
  Mux2/1 -> Mux3/2
  Demux4/1 -> Mux1/1  "vx"
  Mux3/1 -> Out2/1
  Demux4/6 -> Mux2/3  "psi"
  MATLAB Function/1(state_dot) -> Demux4/1
  spec/1 -> MATLAB Function/3(spec)
  state/1 -> MATLAB Function/2(state)

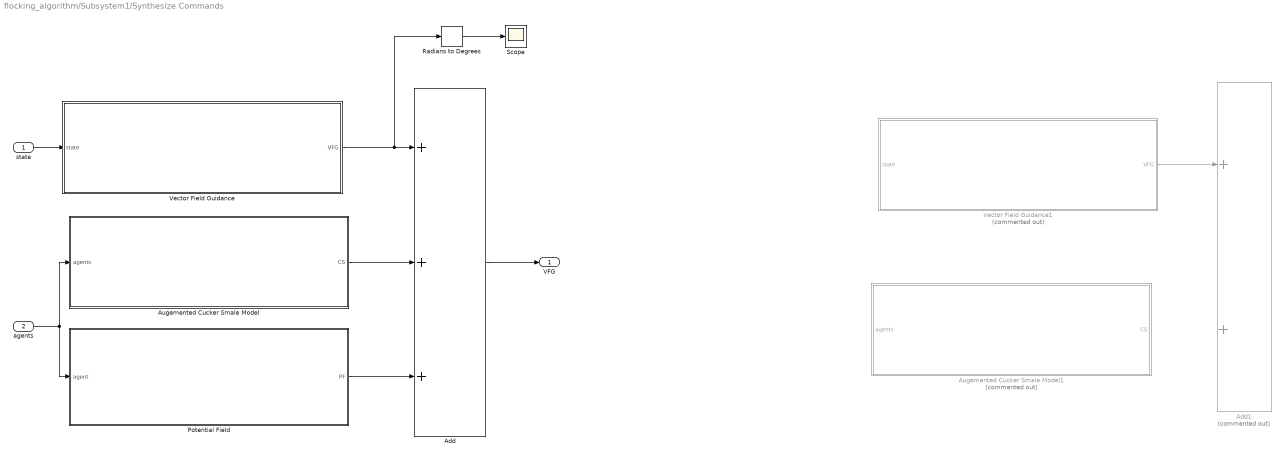
== system flocking_algorithm/Subsystem1/Synthesize Commands ==
  state : Inport
  agents : Inport  Port=2
  Add : Sum  Inputs=+++
  Add1 : Sum  Commented=on
  Augemented Cucker Smale Model : Subsystem
  Augemented Cucker Smale Model1 : Subsystem  Commented=on
  Potential Field : Subsystem
  Radians to Degrees : simulink_extras/Transformations/Radians to Degrees
  Scope : Scope
      settings: ActiveDisplayYMinimum=-3978.1648582066614  ActiveDisplayYMaximum=1014.9954700636738  DataLoggingVariableName=ScopeData2
  Vector Field Guidance : Subsystem
  Vector Field Guidance1 : Subsystem  Commented=on
  VFG : Outport
  wires:
  state/1 -> Vector Field Guidance/1(state)
  Potential Field/1(PF) -> Add/3
  Vector Field Guidance1/1(VFG) -> Add1/1
  Vector Field Guidance/1(VFG) -> Radians to Degrees/1, Add/1
  Radians to Degrees/1 -> Scope/1
  agents/1 -> Augemented Cucker Smale Model/1(agents), Potential Field/1(agent)
  Add/1 -> VFG/1
  Augemented Cucker Smale Model/1(CS) -> Add/2

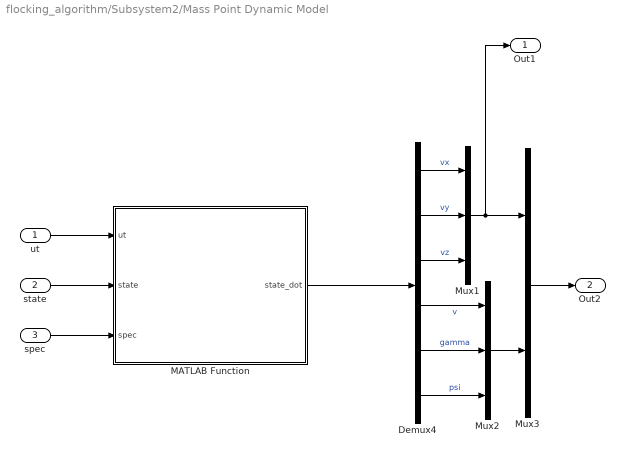
== system flocking_algorithm/Subsystem2/Mass Point Dynamic Model ==
  ut : Inport
  state : Inport  Port=2
  spec : Inport  Port=3
  Demux4 : Demux  Outputs=6
  MATLAB Function : MATLAB Function  TreatAsAtomicUnit=on
  Mux1 : Mux  Inputs=3
  Mux2 : Mux  Inputs=3
  Mux3 : Mux  Inputs=2
  Out1 : Outport
  Out2 : Outport  Port=2
  wires:
  Demux4/5 -> Mux2/2  "gamma"
  Demux4/6 -> Mux2/3  "psi"
  Demux4/4 -> Mux2/1  "v"
  Mux1/1 -> Out1/1, Mux3/1
  Mux2/1 -> Mux3/2
  Demux4/1 -> Mux1/1  "vx"
  Demux4/2 -> Mux1/2  "vy"
  Demux4/3 -> Mux1/3  "vz"
  MATLAB Function/1(state_dot) -> Demux4/1
  Mux3/1 -> Out2/1
  state/1 -> MATLAB Function/2(state)
  ut/1 -> MATLAB Function/1(ut)
  spec/1 -> MATLAB Function/3(spec)

== system flocking_algorithm/Subsystem2/Synthesize Commands ==
  State : Inport
  Agents : Inport  Port=2
  Add : Sum  Inputs=+++
  Augemented Cucker Smale Model : Subsystem
  Potential Field : Subsystem
  Vector Field Guidance : Subsystem
  Out1 : Outport
  wires:
  Vector Field Guidance/1(VFG) -> Add/1
  State/1 -> Vector Field Guidance/1(state)
  Agents/1 -> Augemented Cucker Smale Model/1(agent), Potential Field/1(agent)
  Potential Field/1(PF) -> Add/3
  Add/1 -> Out1/1
  Augemented Cucker Smale Model/1(ACS) -> Add/2

== system flocking_algorithm/Subsystem2/Transform to Autopilot Commands ==
  u_virtual : Inport
  state : Inport  Port=2
  spec : Inport  Port=3
  MATLAB Function : MATLAB Function  TreatAsAtomicUnit=on
  ActualOutput : Outport
  wires:
  u_virtual/1 -> MATLAB Function/1(u_virtual)
  state/1 -> MATLAB Function/2(state)
  spec/1 -> MATLAB Function/3(spec)
  MATLAB Function/1(act_out) -> ActualOutput/1

== system flocking_algorithm/Subsystem3/Mass Point Dynamic Model ==
  ut : Inport
  state : Inport  Port=2
  spec : Inport  Port=3
  Demux4 : Demux  Outputs=6
  MATLAB Function : MATLAB Function  TreatAsAtomicUnit=on
  Mux1 : Mux  Inputs=3
  Mux2 : Mux  Inputs=3
  Mux3 : Mux  Inputs=2
  Out1 : Outport
  Out2 : Outport  Port=2
  wires:
  Demux4/5 -> Mux2/2  "gamma"
  Demux4/6 -> Mux2/3  "psi"
  Demux4/4 -> Mux2/1  "v"
  Mux1/1 -> Out1/1, Mux3/1
  Mux2/1 -> Mux3/2
  Demux4/1 -> Mux1/1  "vx"
  Demux4/2 -> Mux1/2  "vy"
  Demux4/3 -> Mux1/3  "vz"
  MATLAB Function/1(state_dot) -> Demux4/1
  Mux3/1 -> Out2/1
  state/1 -> MATLAB Function/2(state)
  ut/1 -> MATLAB Function/1(ut)
  spec/1 -> MATLAB Function/3(spec)

== system flocking_algorithm/Subsystem3/Synthesize Commands ==
  State : Inport
  Agents : Inport  Port=2
  Add : Sum  Inputs=+++
  Augemented Cucker Smale Model : Subsystem
  Potential Field : Subsystem
  Vector Field Guidance : Subsystem
  Out1 : Outport
  wires:
  Vector Field Guidance/1(VFG) -> Add/1
  State/1 -> Vector Field Guidance/1(state)
  Agents/1 -> Augemented Cucker Smale Model/1(agent), Potential Field/1(agent)
  Potential Field/1(PF) -> Add/3
  Add/1 -> Out1/1
  Augemented Cucker Smale Model/1(ACS) -> Add/2

== system flocking_algorithm/Subsystem3/Transform to Autopilot Commands ==
  u_virtual : Inport
  state : Inport  Port=2
  spec : Inport  Port=3
  MATLAB Function : MATLAB Function  TreatAsAtomicUnit=on
  ActualOutput : Outport
  wires:
  u_virtual/1 -> MATLAB Function/1(u_virtual)
  state/1 -> MATLAB Function/2(state)
  spec/1 -> MATLAB Function/3(spec)
  MATLAB Function/1(act_out) -> ActualOutput/1

== system flocking_algorithm/Subsystem4/Mass Point Dynamic Model ==
  ut : Inport
  state : Inport  Port=2
  spec : Inport  Port=3
  Demux4 : Demux  Outputs=6
  MATLAB Function : MATLAB Function  TreatAsAtomicUnit=on
  Mux1 : Mux  Inputs=3
  Mux2 : Mux  Inputs=3
  Mux3 : Mux  Inputs=2
  Out1 : Outport
  Out2 : Outport  Port=2
  wires:
  Demux4/5 -> Mux2/2  "gamma"
  Demux4/6 -> Mux2/3  "psi"
  Demux4/4 -> Mux2/1  "v"
  Mux1/1 -> Out1/1, Mux3/1
  Mux2/1 -> Mux3/2
  Demux4/1 -> Mux1/1  "vx"
  Demux4/2 -> Mux1/2  "vy"
  Demux4/3 -> Mux1/3  "vz"
  MATLAB Function/1(state_dot) -> Demux4/1
  Mux3/1 -> Out2/1
  state/1 -> MATLAB Function/2(state)
  ut/1 -> MATLAB Function/1(ut)
  spec/1 -> MATLAB Function/3(spec)

== system flocking_algorithm/Subsystem4/Synthesize Commands ==
  State : Inport
  Agents : Inport  Port=2
  Add : Sum  Inputs=+++
  Augemented Cucker Smale Model : Subsystem
  Potential Field : Subsystem
  Vector Field Guidance : Subsystem
  Out1 : Outport
  wires:
  Augemented Cucker Smale Model/1(ACS) -> Add/2
  Agents/1 -> Augemented Cucker Smale Model/1(agent), Potential Field/1(agent)
  Add/1 -> Out1/1
  Potential Field/1(PF) -> Add/3
  Vector Field Guidance/1(VFG) -> Add/1
  State/1 -> Vector Field Guidance/1(state)

== system flocking_algorithm/Subsystem4/Transform to Autopilot Commands ==
  u_virtual : Inport
  state : Inport  Port=2
  spec : Inport  Port=3
  MATLAB Function : MATLAB Function  TreatAsAtomicUnit=on
  ActualOutput : Outport
  wires:
  u_virtual/1 -> MATLAB Function/1(u_virtual)
  state/1 -> MATLAB Function/2(state)
  spec/1 -> MATLAB Function/3(spec)
  MATLAB Function/1(act_out) -> ActualOutput/1

== system flocking_algorithm/Subsystem5/Mass Point Dynamic Model ==
  ut : Inport
  state : Inport  Port=2
  spec : Inport  Port=3
  Demux4 : Demux  Outputs=6
  MATLAB Function : MATLAB Function  TreatAsAtomicUnit=on
  Mux1 : Mux  Inputs=3
  Mux2 : Mux  Inputs=3
  Mux3 : Mux  Inputs=2
  Out1 : Outport
  Out2 : Outport  Port=2
  wires:
  Demux4/5 -> Mux2/2  "gamma"
  Demux4/6 -> Mux2/3  "psi"
  Demux4/4 -> Mux2/1  "v"
  Mux1/1 -> Out1/1, Mux3/1
  Mux2/1 -> Mux3/2
  Demux4/1 -> Mux1/1  "vx"
  Demux4/2 -> Mux1/2  "vy"
  Demux4/3 -> Mux1/3  "vz"
  MATLAB Function/1(state_dot) -> Demux4/1
  Mux3/1 -> Out2/1
  state/1 -> MATLAB Function/2(state)
  ut/1 -> MATLAB Function/1(ut)
  spec/1 -> MATLAB Function/3(spec)

== system flocking_algorithm/Subsystem5/Synthesize Commands ==
  State : Inport
  Agents : Inport  Port=2
  Add : Sum  Inputs=+++
  Augemented Cucker Smale Model : Subsystem
  Potential Field : Subsystem
  Vector Field Guidance : Subsystem
  Out1 : Outport
  wires:
  Augemented Cucker Smale Model/1(ACS) -> Add/2
  Agents/1 -> Augemented Cucker Smale Model/1(agent), Potential Field/1(agent)
  Add/1 -> Out1/1
  Potential Field/1(PF) -> Add/3
  Vector Field Guidance/1(VFG) -> Add/1
  State/1 -> Vector Field Guidance/1(state)

== system flocking_algorithm/Subsystem5/Transform to Autopilot Commands ==
  u_virtual : Inport
  state : Inport  Port=2
  spec : Inport  Port=3
  MATLAB Function : MATLAB Function  TreatAsAtomicUnit=on
  ActualOutput : Outport
  wires:
  u_virtual/1 -> MATLAB Function/1(u_virtual)
  state/1 -> MATLAB Function/2(state)
  spec/1 -> MATLAB Function/3(spec)
  MATLAB Function/1(act_out) -> ActualOutput/1

== system flocking_algorithm/Subsystem/Synthesize Commands/Augemented Cucker Smale Model ==
  agent : Inport
  Add : Sum  Inputs=+++
  Alignment : MATLAB Function  TreatAsAtomicUnit=on
  Repulsion : MATLAB Function  TreatAsAtomicUnit=on
  Scope : Scope  NumInputPorts=4
      settings: ActiveDisplayYMinimum=-0.35686775740168808  ActiveDisplayYMaximum=0.36998625047783196  DataLoggingVariableName=ScopeData4
  Stiffness : MATLAB Function  TreatAsAtomicUnit=on
  ACS : Outport
  wires:
  agent/1 -> Repulsion/1(agent), Stiffness/1(agent), Alignment/1(agent)
  Add/1 -> Scope/4, ACS/1
  Stiffness/1(stiff) -> Scope/2, Add/2
  Alignment/1(align) -> Scope/1, Add/1
  Repulsion/1(rep) -> Scope/3, Add/3

== system flocking_algorithm/Subsystem/Synthesize Commands/Potential Field ==
  agent : Inport
  Potential Field : MATLAB Function  TreatAsAtomicUnit=on
  Scope : Scope
      settings: ActiveDisplayYMinimum=-1.4513538739553342E-6  ActiveDisplayYMaximum=1.2009565479350567E-6  DataLoggingVariableName=ScopeData4
  PF : Outport
  wires:
  agent/1 -> Potential Field/1(agents)
  Potential Field/1(u_pf) -> PF/1, Scope/1

== system flocking_algorithm/Subsystem/Synthesize Commands/Vector Field Guidance2 ==
  state : Inport
  MATLAB Function : MATLAB Function  TreatAsAtomicUnit=on
  Scope : Scope  NumInputPorts=3
      settings: ActiveDisplayYMinimum=-1  ActiveDisplayYMaximum=1  DataLoggingVariableName=ScopeData2
  VFG : Outport
  wires:
  state/1 -> MATLAB Function/1(state)
  MATLAB Function/1(VFG) -> VFG/1
  MATLAB Function/2(psi_wrapped) -> Scope/1
  MATLAB Function/3(des_psi) -> Scope/2
  MATLAB Function/4(psi_err) -> Scope/3

== system flocking_algorithm/Subsystem1/Synthesize Commands/Augemented Cucker Smale Model ==
  agents : Inport
  Add : Sum  Inputs=+++
  Alignment : MATLAB Function  TreatAsAtomicUnit=on
  Repulsion : MATLAB Function  TreatAsAtomicUnit=on
  Scope : Scope  NumInputPorts=4
      settings: ActiveDisplayYMinimum=-0.36922761220470945  ActiveDisplayYMaximum=0.35004001294358511  DataLoggingVariableName=ScopeData6
  Stiffness : MATLAB Function  TreatAsAtomicUnit=on
  CS : Outport
  wires:
  agents/1 -> Repulsion/1(agent), Stiffness/1(agent), Alignment/1(agent)
  Add/1 -> Scope/4, CS/1
  Stiffness/1(stiff) -> Scope/2, Add/2
  Alignment/1(align) -> Scope/1, Add/1
  Repulsion/1(rep) -> Scope/3, Add/3

== system flocking_algorithm/Subsystem1/Synthesize Commands/Augemented Cucker Smale Model1 ==
  agents : Inport
  Add : Sum  Inputs=+++
  Alignment : MATLAB Function  TreatAsAtomicUnit=on
  Alignment1 : MATLAB Function  Commented=on  TreatAsAtomicUnit=on
  Repulsion : MATLAB Function  TreatAsAtomicUnit=on
  Scope : Scope  NumInputPorts=4
      settings: ActiveDisplayYMinimum=-0.36922761220470945  ActiveDisplayYMaximum=0.35004001294358511  DataLoggingVariableName=ScopeData6
  Stiffness : MATLAB Function  TreatAsAtomicUnit=on
  CS : Outport
  wires:
  agents/1 -> Repulsion/1(agent), Stiffness/1(agent), Alignment1/1(agent), Alignment/1(agent)
  Add/1 -> Scope/4, CS/1
  Stiffness/1(stiff) -> Scope/2, Add/2
  Alignment/1(align) -> Scope/1, Add/1
  Repulsion/1(rep) -> Scope/3, Add/3

== system flocking_algorithm/Subsystem1/Synthesize Commands/Potential Field ==
  agent : Inport
  Potential Field : MATLAB Function  TreatAsAtomicUnit=on
  Scope : Scope
      settings: ActiveDisplayYMinimum=-1.5989724044436885E-8  ActiveDisplayYMaximum=1.5989726123536597E-8  DataLoggingVariableName=ScopeData4
  PF : Outport
  wires:
  agent/1 -> Potential Field/1(agents)
  Potential Field/1(u_pf) -> PF/1, Scope/1

== system flocking_algorithm/Subsystem1/Synthesize Commands/Vector Field Guidance ==
  state : Inport
  MATLAB Function : MATLAB Function  TreatAsAtomicUnit=on
  Radians to Degrees : simulink_extras/Transformations/Radians to Degrees
  Radians to Degrees1 : simulink_extras/Transformations/Radians to Degrees
  Radians to Degrees2 : simulink_extras/Transformations/Radians to Degrees
  Scope : Scope  NumInputPorts=3
      settings: ActiveDisplayYMinimum=-388.48504664691143  ActiveDisplayYMaximum=433.05336667048329  DataLoggingVariableName=ScopeData8
  VFG : Outport
  wires:
  MATLAB Function/1(VFG) -> VFG/1
  state/1 -> MATLAB Function/1(state)
  MATLAB Function/2(psi_wrapped) -> Radians to Degrees/1
  MATLAB Function/3(des_psi) -> Radians to Degrees1/1
  Radians to Degrees/1 -> Scope/1  "psi"
  Radians to Degrees1/1 -> Scope/2  "des"
  MATLAB Function/4(psi_err) -> Radians to Degrees2/1
  Radians to Degrees2/1 -> Scope/3  "err"

== system flocking_algorithm/Subsystem1/Synthesize Commands/Vector Field Guidance1 ==
  state : Inport
  Demux : Demux  Outputs=3
  MATLAB Function : MATLAB Function  TreatAsAtomicUnit=on
  Mux : Mux  Inputs=3
  VFG : Outport
  wires:
  Demux/3 -> Mux/3  "uz"
  MATLAB Function/1(VFG) -> Demux/1
  Mux/1 -> VFG/1
  Demux/1 -> Mux/1  "ux"
  Demux/2 -> Mux/2  "uy"
  state/1 -> MATLAB Function/1(state)

== system flocking_algorithm/Subsystem2/Synthesize Commands/Augemented Cucker Smale Model ==
  agent : Inport
  Add : Sum  Inputs=+++
  Alignment : MATLAB Function  TreatAsAtomicUnit=on
  Repulsion : MATLAB Function  TreatAsAtomicUnit=on
  Scope : Scope  NumInputPorts=4
      settings: ActiveDisplayYMinimum=-0.35686775740168808  ActiveDisplayYMaximum=0.36998625047783196  DataLoggingVariableName=ScopeData4
  Stiffness : MATLAB Function  TreatAsAtomicUnit=on
  ACS : Outport
  wires:
  agent/1 -> Repulsion/1(agent), Stiffness/1(agent), Alignment/1(agent)
  Add/1 -> Scope/4, ACS/1
  Stiffness/1(stiff) -> Scope/2, Add/2
  Alignment/1(align) -> Scope/1, Add/1
  Repulsion/1(rep) -> Scope/3, Add/3

== system flocking_algorithm/Subsystem2/Synthesize Commands/Potential Field ==
  agent : Inport
  Potential Field : MATLAB Function  TreatAsAtomicUnit=on
  Scope : Scope
      settings: ActiveDisplayYMinimum=-1.1914624946657111  ActiveDisplayYMaximum=0.13238479012228035  DataLoggingVariableName=ScopeData4
  PF : Outport
  wires:
  agent/1 -> Potential Field/1(agents)
  Potential Field/1(u_pf) -> PF/1, Scope/1

== system flocking_algorithm/Subsystem2/Synthesize Commands/Vector Field Guidance ==
  state : Inport
  MATLAB Function : MATLAB Function  TreatAsAtomicUnit=on
  Scope : Scope  NumInputPorts=3
      settings: ActiveDisplayYMinimum=-1  ActiveDisplayYMaximum=1  DataLoggingVariableName=ScopeData6
  VFG : Outport
  wires:
  MATLAB Function/1(VFG) -> VFG/1
  state/1 -> MATLAB Function/1(state)
  MATLAB Function/2(psi_wrapped) -> Scope/1
  MATLAB Function/3(des_psi) -> Scope/2
  MATLAB Function/4(psi_err) -> Scope/3

== system flocking_algorithm/Subsystem3/Synthesize Commands/Augemented Cucker Smale Model ==
  agent : Inport
  Add : Sum  Inputs=+++
  Alignment : MATLAB Function  TreatAsAtomicUnit=on
  Repulsion : MATLAB Function  TreatAsAtomicUnit=on
  Scope : Scope  NumInputPorts=4
      settings: ActiveDisplayYMinimum=-0.35686775740168808  ActiveDisplayYMaximum=0.36998625047783196  DataLoggingVariableName=ScopeData4
  Stiffness : MATLAB Function  TreatAsAtomicUnit=on
  ACS : Outport
  wires:
  agent/1 -> Repulsion/1(agent), Stiffness/1(agent), Alignment/1(agent)
  Add/1 -> Scope/4, ACS/1
  Stiffness/1(stiff) -> Scope/2, Add/2
  Alignment/1(align) -> Scope/1, Add/1
  Repulsion/1(rep) -> Scope/3, Add/3

== system flocking_algorithm/Subsystem3/Synthesize Commands/Potential Field ==
  agent : Inport
  Potential Field : MATLAB Function  TreatAsAtomicUnit=on
  Scope : Scope
      settings: ActiveDisplayYMinimum=-1.1914624946657111  ActiveDisplayYMaximum=0.13238479012228035  DataLoggingVariableName=ScopeData4
  PF : Outport
  wires:
  agent/1 -> Potential Field/1(agents)
  Potential Field/1(u_pf) -> PF/1, Scope/1

== system flocking_algorithm/Subsystem3/Synthesize Commands/Vector Field Guidance ==
  state : Inport
  MATLAB Function : MATLAB Function  TreatAsAtomicUnit=on
  Scope : Scope  NumInputPorts=3
      settings: DataLoggingVariableName=ScopeData8
  VFG : Outport
  wires:
  state/1 -> MATLAB Function/1(state)
  MATLAB Function/1(VFG) -> VFG/1
  MATLAB Function/2(psi_wrapped) -> Scope/1
  MATLAB Function/3(des_psi) -> Scope/2
  MATLAB Function/4(psi_err) -> Scope/3

== system flocking_algorithm/Subsystem4/Synthesize Commands/Augemented Cucker Smale Model ==
  agent : Inport
  Add : Sum  Inputs=+++
  Alignment : MATLAB Function  TreatAsAtomicUnit=on
  Repulsion : MATLAB Function  TreatAsAtomicUnit=on
  Scope : Scope  NumInputPorts=4
      settings: ActiveDisplayYMinimum=-0.35686775740168808  ActiveDisplayYMaximum=0.36998625047783196  DataLoggingVariableName=ScopeData4
  Stiffness : MATLAB Function  TreatAsAtomicUnit=on
  ACS : Outport
  wires:
  agent/1 -> Repulsion/1(agent), Stiffness/1(agent), Alignment/1(agent)
  Add/1 -> Scope/4, ACS/1
  Stiffness/1(stiff) -> Scope/2, Add/2
  Alignment/1(align) -> Scope/1, Add/1
  Repulsion/1(rep) -> Scope/3, Add/3

== system flocking_algorithm/Subsystem4/Synthesize Commands/Potential Field ==
  agent : Inport
  Potential Field : MATLAB Function  TreatAsAtomicUnit=on
  Scope : Scope
      settings: ActiveDisplayYMinimum=-1.1914624946657111  ActiveDisplayYMaximum=0.13238479012228035  DataLoggingVariableName=ScopeData4
  PF : Outport
  wires:
  agent/1 -> Potential Field/1(agents)
  Potential Field/1(u_pf) -> PF/1, Scope/1

== system flocking_algorithm/Subsystem4/Synthesize Commands/Vector Field Guidance ==
  state : Inport
  MATLAB Function : MATLAB Function  TreatAsAtomicUnit=on
  Scope : Scope  NumInputPorts=3
      settings: ActiveDisplayYMinimum=-1  ActiveDisplayYMaximum=1  DataLoggingVariableName=ScopeData9
  VFG : Outport
  wires:
  MATLAB Function/3(des_psi) -> Scope/2
  state/1 -> MATLAB Function/1(state)
  MATLAB Function/1(VFG) -> VFG/1
  MATLAB Function/4(psi_err) -> Scope/3
  MATLAB Function/2(psi_wrapped) -> Scope/1

== system flocking_algorithm/Subsystem5/Synthesize Commands/Augemented Cucker Smale Model ==
  agent : Inport
  Add : Sum  Inputs=+++
  Alignment : MATLAB Function  TreatAsAtomicUnit=on
  Repulsion : MATLAB Function  TreatAsAtomicUnit=on
  Scope : Scope  NumInputPorts=4
      settings: ActiveDisplayYMinimum=-0.35686775740168808  ActiveDisplayYMaximum=0.36998625047783196  DataLoggingVariableName=ScopeData4
  Stiffness : MATLAB Function  TreatAsAtomicUnit=on
  ACS : Outport
  wires:
  agent/1 -> Repulsion/1(agent), Stiffness/1(agent), Alignment/1(agent)
  Add/1 -> Scope/4, ACS/1
  Stiffness/1(stiff) -> Scope/2, Add/2
  Alignment/1(align) -> Scope/1, Add/1
  Repulsion/1(rep) -> Scope/3, Add/3

== system flocking_algorithm/Subsystem5/Synthesize Commands/Potential Field ==
  agent : Inport
  Potential Field : MATLAB Function  TreatAsAtomicUnit=on
  Scope : Scope
      settings: ActiveDisplayYMinimum=-1.1914624946657111  ActiveDisplayYMaximum=0.13238479012228035  DataLoggingVariableName=ScopeData4
  PF : Outport
  wires:
  agent/1 -> Potential Field/1(agents)
  Potential Field/1(u_pf) -> PF/1, Scope/1

== system flocking_algorithm/Subsystem5/Synthesize Commands/Vector Field Guidance ==
  state : Inport
  MATLAB Function : MATLAB Function  TreatAsAtomicUnit=on
  Scope : Scope  NumInputPorts=3
      settings: ActiveDisplayYMinimum=-1  ActiveDisplayYMaximum=1  DataLoggingVariableName=ScopeData10
  VFG : Outport
  wires:
  MATLAB Function/3(des_psi) -> Scope/2
  state/1 -> MATLAB Function/1(state)
  MATLAB Function/1(VFG) -> VFG/1
  MATLAB Function/4(psi_err) -> Scope/3
  MATLAB Function/2(psi_wrapped) -> Scope/1

== matlab function flocking_algorithm/Subsystem1/Synthesize Commands/Augemented Cucker Smale Model/Repulsion ==
  data: agent input; rep output
function rep = BondingForce2(agent)
    idx     = 2;
    N       = size(agent, 2);
    R       = 75;
    K2      = 0.5; % Bonding gain 2
    pos_i   = agent(1:3, idx);
    acc     = zeros(3,1);
    
    for j = 1:N
        if j == idx, continue; end

        pos_j   = agent(1:3, j);
        r_ij    = norm(pos_i - pos_j);

        if r_ij < 1e-3, r_ij = 1e-3; end
        
        % 2R(150m) 간격을 유지하도록 미는 힘/당기는 힘 계산
        acc     = acc + (K2 / (2 * r_ij)) * (r_ij - 2*R) * (pos_j - pos_i);
    end
    rep = acc;
end

== matlab function flocking_algorithm/Subsystem1/Synthesize Commands/Augemented Cucker Smale Model/Stiffness ==
  data: agent input; stiff output
function stiff = BondingForce1(agent)
    idx     = 2;
    N       = size(agent,2);
    K1      = 0.32; % Bonding gain 1
    pos_i   = agent(1:3, idx);
    vel_i   = agent(4:6, idx);
    acc     = zeros(3,1);
    
    for j = 1:N
        if j == idx, continue; end

        pos_j   = agent(1:3, j);
        rel_pos = pos_i - pos_j;
        rel_vel = vel_i - agent(4:6, j);
        r_ij    = norm(rel_pos);

        if r_ij < 1e-3, r_ij = 1e-3; end
        
        % Inner Product
        dot_val = dot(rel_vel, rel_pos);
        acc     = acc + (K1 / (2 * r_ij^2)) * dot_val * (pos_j - pos_i);
    end
    stiff = acc;
end

== matlab function flocking_algorithm/Subsystem1/Synthesize Commands/Potential Field/Potential Field ==
  data: agents input; u_pf output
function u_pf = PF(agents)

    %% params
    idx = 2;
    N = size(agents,2);
    alp = 5*sqrt(2); % Potential Strength
    % Bell Function Constant (a, b, c)
    a   = 75; 
    b   = 4;
    c   = 0;
    sum = zeros(3,1);

    % Agent Information
    pos_i = agents(1:3,idx);

    for j = 1: N
        if idx==j 
            continue; 
        end
        pos_j = agents(1:3, j);
        pos_ij = pos_i - pos_j;
        norm_ij = norm(pos_ij);

        val = (norm_ij - c)/a;
        denominator = 1 + (abs(val))^(2*b);
        if norm_ij > 0.001
            sum = sum + (alp/denominator)*(pos_ij/norm_ij);
        end
    end
    u_pf = sum;
end
